simulink model "sst_llc_npc_inv"  (R2025b)
settings: Solver=ode23tb  StartTime=0.0  StopTime=simlength  FixedStep=tc  MaxStep=tc
values from neighbouring files (symbols this model uses):
  Adrso = eye(2) + Arso*ts_inv    [init_model.m]
  Aresd_max = eye(2) + Ares_max*ts_afe    [init_model.m]
  Aresd_min = eye(2) + Ares_min*ts_afe    [init_model.m]
  Aresd_nom = eye(2) + Ares_nom*ts_afe    [init_model.m]
  Bresd = Bres*ts_afe    [init_model.m]
  CFi_dc2 = 900e-6*4    (= 0.0036)    [init_model.m]
  Cresd = Cres    [init_model.m]
  Crso = [1 0]    [init_model.m]
  delta = 0.025    [init_model.m]
  fPWM_DAB = fPWM*4    (= 20000)    [init_model.m]
  freq = 50    [init_model.m]
  Iac_FS = I_phase_normalization_factor    [init_model.m]
  Idc_FS = max(Idab1_dc_nom,Idab2_dc_nom) * margin_factor    [init_model.m]
  iph_grid_pu_ref = 3.75    [init_model.m]
  ki_afe = 18    [init_model.m]
  ki_i_dab = 18    [init_model.m]
  ki_pll = 3140    [init_model.m]
  ki_rpi = 18    [init_model.m]
  kp_afe = 0.25    [init_model.m]
  kp_i_dab = 0.25    [init_model.m]
  kp_pll = 314    [init_model.m]
  kp_rpi = 0.25    [init_model.m]
  Ldrso = acker(Adrso',Crso',polesdrso)'    [init_model.m]
  LFu1_AFE = 0.33e-3    (= 0.00033)    [init_model.m]
  n_modules = 1    [init_model.m]
  RLFu1_AFE = 157*0.05*LFu1_AFE    (= 0.0025905)    [init_model.m]
  tc = ts_dab/1000*24    (= 1.2e-06)    [init_model.m]
  ts_afe = 1/fPWM_AFE    (= 0.0002)    [init_model.m]
  ts_dab = 1/fPWM_DAB    (= 5e-05)    [init_model.m]
  ts_inv = 1/fPWM_INV    (= 0.0002)    [init_model.m]
  Vac_FS = V_phase_normalization_factor    [init_model.m]
  Vdab2_dc_nom = 1500    [init_model.m]
  Vdc_FS = max(Vdab1_dc_nom,Vdab2_dc_nom) * margin_factor    [init_model.m]
undefined symbols (not defined in the file or in its folder): omega_grid_nom, V_phase_normalization_factor
libraries: fl_lib x68, nesl_utility x40, discrete_time_low_pass_filter x4, full_bridge_mosfet_based_with_thermal_model x2, single_phase_transformer x2, pi_ctrl x2, resonant_llc_modulator x2, full_bridge_ideal_switch x2, dclink_for_three_levels x2, full_bridge_three_level_npc_ideal_switch_based_model x2, single_phase_three_levels_PWM_modulator x2, dq_vector_pi x2
(part 2 of 4)

== system sst_llc_npc_inv/global timing/time_afe1 ==
  correction_time : Inport
  Constant : Constant
  Gain : Gain  Gain=k
  Product : Product
  Sum : Sum  Inputs=|++
  time_1 : Clock
  Out1 : Outport
  wires:
  time_1/1 -> Gain/1
  Gain/1 -> Product/1
  Product/1 -> Out1/1
  correction_time/1 -> Sum/1
  Sum/1 -> Product/2
  Constant/1 -> Sum/2

== system sst_llc_npc_inv/global timing/time_afe2 ==
  correction_time : Inport
  Constant : Constant
  Gain : Gain  Gain=k
  Product : Product
  Sum : Sum  Inputs=|++
  time_1 : Clock
  Out1 : Outport
  wires:
  time_1/1 -> Gain/1
  Gain/1 -> Product/1
  Product/1 -> Out1/1
  correction_time/1 -> Sum/1
  Constant/1 -> Sum/2
  Sum/1 -> Product/2

== system sst_llc_npc_inv/global timing/time_afe3 ==
  Gain : Gain  Gain=k
  time_1 : Clock
  Out1 : Outport
  wires:
  Gain/1 -> Out1/1
  time_1/1 -> Gain/1

== system sst_llc_npc_inv/global timing/time_inv1 ==
  correction_time : Inport
  Constant : Constant
  Gain : Gain  Gain=k
  Product : Product
  Sum : Sum  Inputs=|++
  time_1 : Clock
  Out1 : Outport
  wires:
  time_1/1 -> Gain/1
  Gain/1 -> Product/1
  Product/1 -> Out1/1
  correction_time/1 -> Sum/1
  Constant/1 -> Sum/2
  Sum/1 -> Product/2

== system sst_llc_npc_inv/global timing/time_inv2 ==
  correction_time : Inport
  Constant : Constant
  Gain : Gain  Gain=k
  Product : Product
  Sum : Sum  Inputs=|++
  time_1 : Clock
  Out1 : Outport
  wires:
  time_1/1 -> Gain/1
  Gain/1 -> Product/1
  Product/1 -> Out1/1
  correction_time/1 -> Sum/1
  Constant/1 -> Sum/2
  Sum/1 -> Product/2

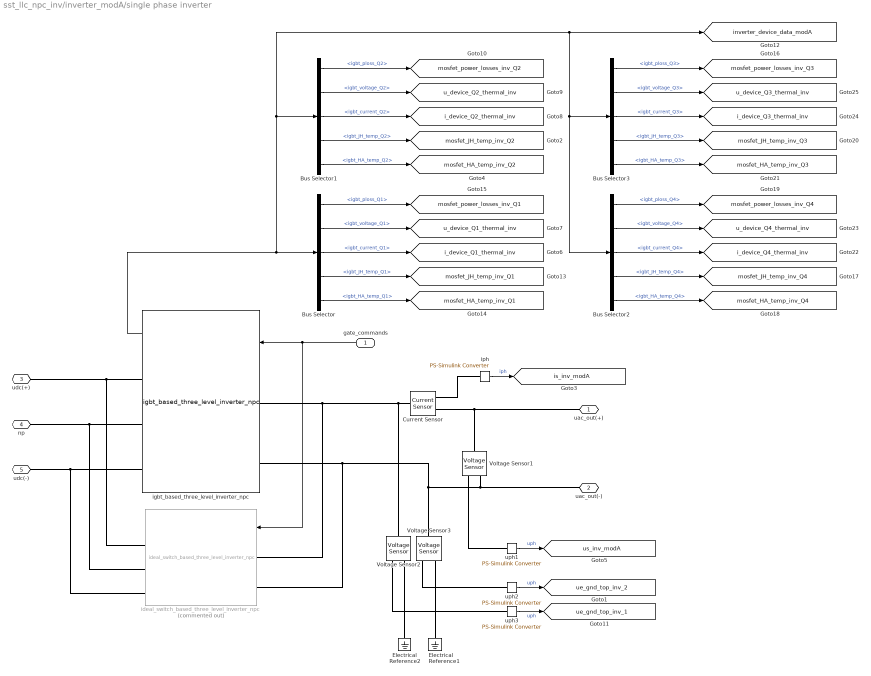
== system sst_llc_npc_inv/inverter_modA/single phase inverter ==
  gate_commands : Inport
  Bus Selector : BusSelector  OutputSignals=igbt_ploss_Q1,igbt_voltage_Q1,igbt_current_Q1,igbt_JH_temp_Q1,igbt_HA_temp_Q1
  Bus Selector1 : BusSelector  OutputSignals=igbt_ploss_Q2,igbt_voltage_Q2,igbt_current_Q2,igbt_JH_temp_Q2,igbt_HA_temp_Q2
  Bus Selector2 : BusSelector  OutputSignals=igbt_ploss_Q4,igbt_voltage_Q4,igbt_current_Q4,igbt_JH_temp_Q4,igbt_HA_temp_Q4
  Bus Selector3 : BusSelector  OutputSignals=igbt_ploss_Q3,igbt_voltage_Q3,igbt_current_Q3,igbt_JH_temp_Q3,igbt_HA_temp_Q3
  Current Sensor : fl_lib/Electrical/Electrical Sensors/Current Sensor
  Electrical Reference1 : fl_lib/Electrical/Electrical Elements/Electrical Reference
  Electrical Reference2 : fl_lib/Electrical/Electrical Elements/Electrical Reference
  Voltage Sensor1 : fl_lib/Electrical/Electrical Sensors/Voltage Sensor
  Voltage Sensor2 : fl_lib/Electrical/Electrical Sensors/Voltage Sensor
  Voltage Sensor3 : fl_lib/Electrical/Electrical Sensors/Voltage Sensor
  ideal_switch_based_three_level_inverter_npc : full_bridge_three_level_npc_ideal_switch_based_model/ideal_switch_based_three_level_inverter_npc  Commented=on  Vth=5.5  Ron=1.5e-3  Vdon_diode=1.65  Rdon_diode=0.15e-3  Csnubber=1e-10  Rsnubber=2200
  igbt_based_three_level_inverter_npc : full_bridge_three_level_npc_igbt_based_model/igbt_based_three_level_inverter_npc  Vth=inv.Vth  Vce_sat=inv.Vce_sat  Rce_on=inv.Rce_on  Eon=inv.Eon  Eoff=inv.Eoff  Erec=inv.Erec  Ion_sw_loss=inv.Ion_sw_losses  Voff_sw_loss=inv.Voff_sw_losses  Vdon_diode=inv.Vdon_diode  Rdon_diode=inv.Rdon_diode  rth_mosfet_JH=inv.Rth_switch_JH  rth_mosfet_HA=Rth_switch_HA  Csnubber=inv.Csnubber  Rsnubber=inv.Rsnubber  JunctionTermalMass=JunctionTermalMass  mass_heatsink=weigth  specific_heat=cp_al  Tambient=Tambient  DThs_init=DThs_init  tc=tc
  iph : nesl_utility/PS-Simulink Converter  PhysicalDomain=network_engine_domain  SubClassName=ps_output  LeftPortType=input  RightPortType=output  PseudoPeriodic=off  Frequencies=[]  VectorFormat=1-D array  Unit=A  AffineConversion=off
  uph1 : nesl_utility/PS-Simulink Converter  PhysicalDomain=network_engine_domain  SubClassName=ps_output  LeftPortType=input  RightPortType=output  PseudoPeriodic=off  Frequencies=[]  VectorFormat=1-D array  Unit=V  AffineConversion=off
  uph2 : nesl_utility/PS-Simulink Converter  PhysicalDomain=network_engine_domain  SubClassName=ps_output  LeftPortType=input  RightPortType=output  PseudoPeriodic=off  Frequencies=[]  VectorFormat=1-D array  Unit=V  AffineConversion=off
  uph3 : nesl_utility/PS-Simulink Converter  PhysicalDomain=network_engine_domain  SubClassName=ps_output  LeftPortType=input  RightPortType=output  PseudoPeriodic=off  Frequencies=[]  VectorFormat=1-D array  Unit=V  AffineConversion=off
  uac_out(+) : PMIOPort  Side=Left
  uac_out(-) : PMIOPort  Port=2  Side=Left
  udc(+) : PMIOPort  Port=3  Side=Right
  np : PMIOPort  Port=4  Side=Right
  udc(-) : PMIOPort  Port=5  Side=Right
  tag scope: i_device_Q1_thermal_inv=global, i_device_Q2_thermal_inv=global, i_device_Q3_thermal_inv=global, i_device_Q4_thermal_inv=global, inverter_device_data_modA=global, is_inv_modA=global, mosfet_HA_temp_inv_Q1=global, mosfet_HA_temp_inv_Q2=global, mosfet_HA_temp_inv_Q3=global, mosfet_HA_temp_inv_Q4=global, mosfet_JH_temp_inv_Q1=global, mosfet_JH_temp_inv_Q2=global, mosfet_JH_temp_inv_Q3=global, mosfet_JH_temp_inv_Q4=global, mosfet_power_losses_inv_Q1=global, mosfet_power_losses_inv_Q2=global, mosfet_power_losses_inv_Q3=global, mosfet_power_losses_inv_Q4=global, u_device_Q1_thermal_inv=global, u_device_Q2_thermal_inv=global, u_device_Q3_thermal_inv=global, u_device_Q4_thermal_inv=global, ue_gnd_top_inv_1=global, ue_gnd_top_inv_2=global, us_inv_modA=global
  wires:
  iph/1 -> [is_inv_modA]  "iph"
  uph1/1 -> [us_inv_modA]  "uph"
  gate_commands/1 -> ideal_switch_based_three_level_inverter_npc/1, igbt_based_three_level_inverter_npc/1
  Bus Selector/1 -> [mosfet_power_losses_inv_Q1]  "<igbt_ploss_Q1>"
  Bus Selector/2 -> [u_device_Q1_thermal_inv]  "<igbt_voltage_Q1>"
  Bus Selector/3 -> [i_device_Q1_thermal_inv]  "<igbt_current_Q1>"
  Bus Selector/4 -> [mosfet_JH_temp_inv_Q1]  "<igbt_JH_temp_Q1>"
  Bus Selector/5 -> [mosfet_HA_temp_inv_Q1]  "<igbt_HA_temp_Q1>"
  Bus Selector1/4 -> [mosfet_JH_temp_inv_Q2]  "<igbt_JH_temp_Q2>"
  Bus Selector1/5 -> [mosfet_HA_temp_inv_Q2]  "<igbt_HA_temp_Q2>"
  Bus Selector1/3 -> [i_device_Q2_thermal_inv]  "<igbt_current_Q2>"
  Bus Selector1/2 -> [u_device_Q2_thermal_inv]  "<igbt_voltage_Q2>"
  Bus Selector1/1 -> [mosfet_power_losses_inv_Q2]  "<igbt_ploss_Q2>"
  uph2/1 -> [ue_gnd_top_inv_2]  "uph"
  uph3/1 -> [ue_gnd_top_inv_1]  "uph"
  igbt_based_three_level_inverter_npc/1 -> Bus Selector2/1, Bus Selector3/1, [inverter_device_data_modA], Bus Selector1/1, Bus Selector/1
  Bus Selector3/1 -> [mosfet_power_losses_inv_Q3]  "<igbt_ploss_Q3>"
  Bus Selector3/2 -> [u_device_Q3_thermal_inv]  "<igbt_voltage_Q3>"
  Bus Selector3/3 -> [i_device_Q3_thermal_inv]  "<igbt_current_Q3>"
  Bus Selector3/5 -> [mosfet_HA_temp_inv_Q3]  "<igbt_HA_temp_Q3>"
  Bus Selector3/4 -> [mosfet_JH_temp_inv_Q3]  "<igbt_JH_temp_Q3>"
  Bus Selector2/5 -> [mosfet_HA_temp_inv_Q4]  "<igbt_HA_temp_Q4>"
  Bus Selector2/4 -> [mosfet_JH_temp_inv_Q4]  "<igbt_JH_temp_Q4>"
  Bus Selector2/3 -> [i_device_Q4_thermal_inv]  "<igbt_current_Q4>"
  Bus Selector2/2 -> [u_device_Q4_thermal_inv]  "<igbt_voltage_Q4>"
  Bus Selector2/1 -> [mosfet_power_losses_inv_Q4]  "<igbt_ploss_Q4>"
  connections:
  Current Sensor/RConn1 -- iph/LConn1
  Current Sensor/RConn2 -- Voltage Sensor1/LConn1 -- uac_out(+)/RConn1
  Voltage Sensor1/RConn1 -- uph1/LConn1
  Voltage Sensor1/RConn2 -- ideal_switch_based_three_level_inverter_npc/LConn2 -- igbt_based_three_level_inverter_npc/LConn2 -- Voltage Sensor3/LConn1 -- uac_out(-)/RConn1
  igbt_based_three_level_inverter_npc/RConn1 -- ideal_switch_based_three_level_inverter_npc/RConn1 -- udc(+)/RConn1
  Current Sensor/LConn1 -- ideal_switch_based_three_level_inverter_npc/LConn1 -- igbt_based_three_level_inverter_npc/LConn1 -- Voltage Sensor2/LConn1
  igbt_based_three_level_inverter_npc/RConn3 -- ideal_switch_based_three_level_inverter_npc/RConn3 -- udc(-)/RConn1
  Electrical Reference2/LConn1 -- Voltage Sensor2/RConn2
  Electrical Reference1/LConn1 -- Voltage Sensor3/RConn2
  uph2/LConn1 -- Voltage Sensor3/RConn1
  uph3/LConn1 -- Voltage Sensor2/RConn1
  igbt_based_three_level_inverter_npc/RConn2 -- ideal_switch_based_three_level_inverter_npc/RConn2 -- np/RConn1

== system sst_llc_npc_inv/inverter_modA/single phase inverter control1 ==
  Constant : Constant
  acquisition_and_scaling_current : Subsystem
  acquisition_and_scaling_dc_voltage : Subsystem
  acquisition_and_scaling_voltage : Subsystem
  acquisition_and_scaling_voltage1 : Subsystem
  inverter_current_output_pu_reference : Subsystem
  pwm modulator : Subsystem
  rpi_based_single_phase_inverter_ctrl : Subsystem
  gate_cmds : Outport
  u_ctrl_out : Outport  Port=2
  tag scope: phase_synch_modA=global
  wires:
  [is_inv_modA] -> acquisition_and_scaling_current/1(in)
  pwm modulator/1(gate_cmds) -> gate_cmds/1
  [TRGO_INV_1] -> rpi_based_single_phase_inverter_ctrl/Trigger
  [inverter_voltage_output_modA] -> acquisition_and_scaling_voltage/1(in)
  acquisition_and_scaling_current/1(out) -> rpi_based_single_phase_inverter_ctrl/2(is_inv_pu)  "is_inv_pu"
  acquisition_and_scaling_voltage/1(out) -> rpi_based_single_phase_inverter_ctrl/1(inverter_voltage_output_pu)  "inverter_voltage_output_pu"
  inverter_current_output_pu_reference/1(inverter_current_output_pu_reference) -> rpi_based_single_phase_inverter_ctrl/3(is_inv_pu_reference)  "inverter_current_output_pu_reference"
  [dclink_voltage_inverter_modA] -> acquisition_and_scaling_dc_voltage/1(in)
  rpi_based_single_phase_inverter_ctrl/1(u_ctrl_out) -> u_ctrl_out/1, pwm modulator/1(vout)
  acquisition_and_scaling_voltage1/1(out) -> rpi_based_single_phase_inverter_ctrl/5(u_line_pu)  "ac_grid_voltage_pu"
  [ac_grid_voltage] -> acquisition_and_scaling_voltage1/1(in)
  rpi_based_single_phase_inverter_ctrl/2(phase_grid_modA) -> [phase_synch_modA]
  [time_afe_module_1] -> rpi_based_single_phase_inverter_ctrl/6(time_afe_module_1)  "time_afe_module_1"
  Constant/1 -> rpi_based_single_phase_inverter_ctrl/4(dclink_voltage_pu)

== system sst_llc_npc_inv/inverter_modB/single phase inverter ==
  gate_commands : Inport
  Bus Selector : BusSelector  OutputSignals=switch_voltage_Q1,switch_current_Q1
  Current Sensor : fl_lib/Electrical/Electrical Sensors/Current Sensor
  Electrical Reference1 : fl_lib/Electrical/Electrical Elements/Electrical Reference
  Electrical Reference2 : fl_lib/Electrical/Electrical Elements/Electrical Reference
  Voltage Sensor1 : fl_lib/Electrical/Electrical Sensors/Voltage Sensor
  Voltage Sensor2 : fl_lib/Electrical/Electrical Sensors/Voltage Sensor
  Voltage Sensor3 : fl_lib/Electrical/Electrical Sensors/Voltage Sensor
  ideal_switch_based_three_level_inverter_npc : full_bridge_three_level_npc_ideal_switch_based_model/ideal_switch_based_three_level_inverter_npc  Vth=5.5  Ron=1.5e-3  Vdon_diode=1.65  Rdon_diode=0.15e-3  Csnubber=1e-10  Rsnubber=2200
  iph : nesl_utility/PS-Simulink Converter  PhysicalDomain=network_engine_domain  SubClassName=ps_output  LeftPortType=input  RightPortType=output  PseudoPeriodic=off  Frequencies=[]  VectorFormat=1-D array  Unit=A  AffineConversion=off
  uph1 : nesl_utility/PS-Simulink Converter  PhysicalDomain=network_engine_domain  SubClassName=ps_output  LeftPortType=input  RightPortType=output  PseudoPeriodic=off  Frequencies=[]  VectorFormat=1-D array  Unit=V  AffineConversion=off
  uph2 : nesl_utility/PS-Simulink Converter  PhysicalDomain=network_engine_domain  SubClassName=ps_output  LeftPortType=input  RightPortType=output  PseudoPeriodic=off  Frequencies=[]  VectorFormat=1-D array  Unit=V  AffineConversion=off
  uph3 : nesl_utility/PS-Simulink Converter  PhysicalDomain=network_engine_domain  SubClassName=ps_output  LeftPortType=input  RightPortType=output  PseudoPeriodic=off  Frequencies=[]  VectorFormat=1-D array  Unit=V  AffineConversion=off
  uac_out(+) : PMIOPort  Side=Left
  uac_out(-) : PMIOPort  Port=2  Side=Left
  udc(+) : PMIOPort  Port=3  Side=Right
  np : PMIOPort  Port=4  Side=Right
  udc(-) : PMIOPort  Port=5  Side=Right
  tag scope: i_device_Q1_ideal_inv_modB=global, inverter_device_data_modB=global, is_inv_modB=global, u_device_Q1_ideal_inv_modB=global, ue_gnd_bottom_inv_1=global, ue_gnd_bottom_inv_2=global, us_inv_modB=global
  wires:
  gate_commands/1 -> ideal_switch_based_three_level_inverter_npc/1
  uph1/1 -> [us_inv_modB]  "uph"
  iph/1 -> [is_inv_modB]  "iph"
  uph3/1 -> [ue_gnd_bottom_inv_1]  "uph"
  uph2/1 -> [ue_gnd_bottom_inv_2]  "uph"
  ideal_switch_based_three_level_inverter_npc/1 -> Bus Selector/1, [inverter_device_data_modB]
  Bus Selector/2 -> [i_device_Q1_ideal_inv_modB]  "<switch_current_Q1>"
  Bus Selector/1 -> [u_device_Q1_ideal_inv_modB]  "<switch_voltage_Q1>"
  connections:
  ideal_switch_based_three_level_inverter_npc/RConn3 -- udc(-)/RConn1
  Voltage Sensor2/LConn1 -- ideal_switch_based_three_level_inverter_npc/LConn1 -- Current Sensor/LConn1
  ideal_switch_based_three_level_inverter_npc/RConn1 -- udc(+)/RConn1
  uac_out(-)/RConn1 -- ideal_switch_based_three_level_inverter_npc/LConn2 -- Voltage Sensor3/LConn1 -- Voltage Sensor1/RConn2
  Voltage Sensor1/RConn1 -- uph1/LConn1
  uac_out(+)/RConn1 -- Voltage Sensor1/LConn1 -- Current Sensor/RConn2
  Current Sensor/RConn1 -- iph/LConn1
  Electrical Reference2/LConn1 -- Voltage Sensor2/RConn2
  uph2/LConn1 -- Voltage Sensor3/RConn1
  uph3/LConn1 -- Voltage Sensor2/RConn1
  Electrical Reference1/LConn1 -- Voltage Sensor3/RConn2
  ideal_switch_based_three_level_inverter_npc/RConn2 -- np/RConn1

== system sst_llc_npc_inv/inverter_modB/single phase inverter control1 ==
  acquisition_and_scaling_current : Subsystem
  acquisition_and_scaling_dc_voltage : Subsystem
  acquisition_and_scaling_voltage : Subsystem
  acquisition_and_scaling_voltage1 : Subsystem
  inverter_current_output_pu_reference : Subsystem
  pwm modulator : Subsystem
  rpi_based_single_phase_inverter_ctrl : Subsystem
  gate_cmds : Outport
  tag scope: phase_synch_modB=global
  wires:
  pwm modulator/1(gate_cmds) -> gate_cmds/1
  rpi_based_single_phase_inverter_ctrl/2(phase_grid_modA) -> [phase_synch_modB]
  rpi_based_single_phase_inverter_ctrl/1(u_ctrl_out) -> pwm modulator/1(vout)
  [u_ctrl_out_master] -> rpi_based_single_phase_inverter_ctrl/6(u_ctrl_out_master)  "u_ctrl_out_master"
  acquisition_and_scaling_dc_voltage/1(out) -> rpi_based_single_phase_inverter_ctrl/4(dclink_voltage_pu)
  acquisition_and_scaling_voltage1/1(out) -> rpi_based_single_phase_inverter_ctrl/5(u_line_pu)  "u_line_pu"
  acquisition_and_scaling_current/1(out) -> rpi_based_single_phase_inverter_ctrl/2(is_inv_pu)  "is_inv_pu"
  [inverter_voltage_output_modB] -> acquisition_and_scaling_voltage/1(in)
  [ac_grid_voltage] -> acquisition_and_scaling_voltage1/1(in)
  acquisition_and_scaling_voltage/1(out) -> rpi_based_single_phase_inverter_ctrl/1(inverter_voltage_output_pu)  "inverter_voltage_output_pu"
  [dclink_voltage_inverter_modB] -> acquisition_and_scaling_dc_voltage/1(in)
  [is_inv_modB] -> acquisition_and_scaling_current/1(in)
  inverter_current_output_pu_reference/1(inverter_current_output_pu_reference) -> rpi_based_single_phase_inverter_ctrl/3(is_inv_pu_reference)  "inverter_current_output_pu_reference"
  [TRGO_INV_2] -> rpi_based_single_phase_inverter_ctrl/Trigger

== system sst_llc_npc_inv/line_source/phase_gen ==
  Constant4 : Constant  Value=50*2*pi
  Integrator : Integrator
  bounder1 : MATLAB Function  TreatAsAtomicUnit=on
  phase_gen : Outport  VectorParamsAs1DForOutWhenUnconnected=off
  wires:
  Constant4/1 -> Integrator/1
  Integrator/1 -> bounder1/1(u)
  bounder1/1(y) -> phase_gen/1  "grid_emu_phase"

== system sst_llc_npc_inv/scopes/scopes_dab_modA ==
  Bus Selector : BusSelector  OutputSignals=mosfet_ploss_Q1,mosfet_ploss_Q2
  Bus Selector1 : BusSelector  OutputSignals=mosfet_ploss_Q1,mosfet_ploss_Q2
  dab TR i2/i1 modA : Scope  NumInputPorts=2
      settings: SampleTime=tc  ActiveDisplayYMinimum=-1515.8601129634949  ActiveDisplayYMaximum=1519.4045908602914  DataLoggingVariableName=ScopeData13
  dab TR u2/u1 modA : Scope  NumInputPorts=2
      settings: SampleTime=tc  ActiveDisplayYMinimum=-893.62031856834165  ActiveDisplayYMaximum=653.92363611228757  DataLoggingVariableName=ScopeData4
  dab current output/input modA : Scope  NumInputPorts=2
      settings: SampleTime=tc  ActiveDisplayYMinimum=-34.407086049322743  ActiveDisplayYMaximum=284.20809963586862  DataLoggingVariableName=ScopeData8
  dab outputs modA : Scope  NumInputPorts=2
      settings: SampleTime=tc  ActiveDisplayYMinimum=-1504.2584903012705  ActiveDisplayYMaximum=905.23681286440785  DataLoggingVariableName=ScopeData6
  dab voltage input/output modA : Scope  NumInputPorts=2
      settings: SampleTime=tc  ActiveDisplayYMinimum=-224.45374462345234  ActiveDisplayYMaximum=1977.0471198962268  DataLoggingVariableName=ScopeData10
  dab_analysis_modA : Scope  NumInputPorts=4
      settings: SampleTime=tc  ActiveDisplayYMinimum=-1467.7661945335567  ActiveDisplayYMaximum=1564.8120287034021  DataLoggingVariableName=ScopeData15
  dab_analysis_power loss : Scope  NumInputPorts=4
      settings: SampleTime=tc  ActiveDisplayYMinimum=-26.281609666205206  ActiveDisplayYMaximum=283.03149514655593  DataLoggingVariableName=ScopeData17
  wires:
  [dab_voltage_input_modA] -> dab voltage input/output modA/1  "dab_voltage_input_modA"
  [dab_current_output_modA] -> dab current output/input modA/1  "dab_current_output_modA"
  [dab_voltage_output_modA] -> dab voltage input/output modA/2  "dab_voltage_output_modA"
  [dab_current_input_modA] -> dab current output/input modA/2  "dab_current_input_modA"
  [i2_dab_transformer_modA] -> dab TR i2/i1 modA/1  "i2_dab_transformer_modA"
  [i1_dab_transformer_modA] -> dab TR i2/i1 modA/2  "i1_dab_transformer_modA"
  [u2_dab_transformer_modA] -> dab TR u2/u1 modA/1  "u2_dab_transformer_modA"
  [u1_dab_transformer_modA] -> dab TR u2/u1 modA/2  "u1_dab_transformer_modA"
  [dab_voltage_output_modA] -> dab outputs modA/2  "dab_voltage_output_modA"
  [dab_current_output_modA] -> dab outputs modA/1  "dab_current_output_modA"
  [i2_dab_transformer_modA] -> dab_analysis_modA/1  "i2_dab_transformer_modA"
  [i1_dab_transformer_modA] -> dab_analysis_modA/2  "i1_dab_transformer_modA"
  [u1_dab_transformer_modA] -> dab_analysis_modA/3  "u1_dab_transformer_modA"
  [u2_dab_transformer_modA] -> dab_analysis_modA/4  "u2_dab_transformer_modA"
  [inverter_1_dab_devices_modA] -> Bus Selector/1
  [inverter_2_dab_devices_modA] -> Bus Selector1/1
  Bus Selector/1 -> dab_analysis_power loss/1  "<mosfet_ploss_Q1>"
  Bus Selector/2 -> dab_analysis_power loss/2  "<mosfet_ploss_Q2>"
  Bus Selector1/1 -> dab_analysis_power loss/3  "<mosfet_ploss_Q1>"
  Bus Selector1/2 -> dab_analysis_power loss/4  "<mosfet_ploss_Q2>"

== system sst_llc_npc_inv/scopes/scopes_dab_modB ==
  dab TR i2/i1 modB : Scope  NumInputPorts=2
      settings: SampleTime=tc  ActiveDisplayYMinimum=-700.08630880673149  ActiveDisplayYMaximum=469.74027472719069  DataLoggingVariableName=ScopeData13
  dab TR u2/u1 modB : Scope  NumInputPorts=2
      settings: SampleTime=tc  ActiveDisplayYMinimum=-893.62031856834165  ActiveDisplayYMaximum=653.92363611228757  DataLoggingVariableName=ScopeData4
  dab current output/input modB : Scope  NumInputPorts=2
      settings: SampleTime=tc  ActiveDisplayYMinimum=-7335.7913745283768  ActiveDisplayYMaximum=23819.434208451414  DataLoggingVariableName=ScopeData8
  dab outputs modB : Scope  NumInputPorts=2
      settings: SampleTime=tc  ActiveDisplayYMinimum=-1276.7812228163118  ActiveDisplayYMaximum=1202.3221787513703  DataLoggingVariableName=ScopeData6
  dab voltage input/output modB : Scope  NumInputPorts=2
      settings: SampleTime=tc  ActiveDisplayYMinimum=-237.60937353263552  ActiveDisplayYMaximum=2138.4843617937204  DataLoggingVariableName=ScopeData10
  dab_analysis_modB : Scope  NumInputPorts=4
      settings: SampleTime=tc  ActiveDisplayYMinimum=-1515.8601129634949  ActiveDisplayYMaximum=1519.4045908602914  DataLoggingVariableName=ScopeData15
  wires:
  [u2_dab_transformer_modB] -> dab_analysis_modB/4  "u2_dab_transformer_modB"
  [u1_dab_transformer_modB] -> dab_analysis_modB/3  "u1_dab_transformer_modB"
  [i1_dab_transformer_modB] -> dab_analysis_modB/2  "i1_dab_transformer_modB"
  [i2_dab_transformer_modB] -> dab_analysis_modB/1  "i2_dab_transformer_modB"
  [dab_current_output_modB] -> dab outputs modB/1  "dab_current_output_modB"
  [dab_voltage_output_modB] -> dab outputs modB/2  "dab_voltage_output_modB"
  [u1_dab_transformer_modB] -> dab TR u2/u1 modB/2  "u1_dab_transformer_modB"
  [u2_dab_transformer_modB] -> dab TR u2/u1 modB/1  "u2_dab_transformer_modB"
  [i1_dab_transformer_modB] -> dab TR i2/i1 modB/2  "i1_dab_transformer_modB"
  [i2_dab_transformer_modB] -> dab TR i2/i1 modB/1  "i2_dab_transformer_modB"
  [dab_current_input_modB] -> dab current output/input modB/2  "dab_current_input_modB"
  [dab_voltage_output_modB] -> dab voltage input/output modB/2  "dab_voltage_output_modB"
  [dab_current_output_modB] -> dab current output/input modB/1  "dab_current_output_modB"
  [dab_voltage_input_modB] -> dab voltage input/output modB/1  "dab_voltage_input_modB"

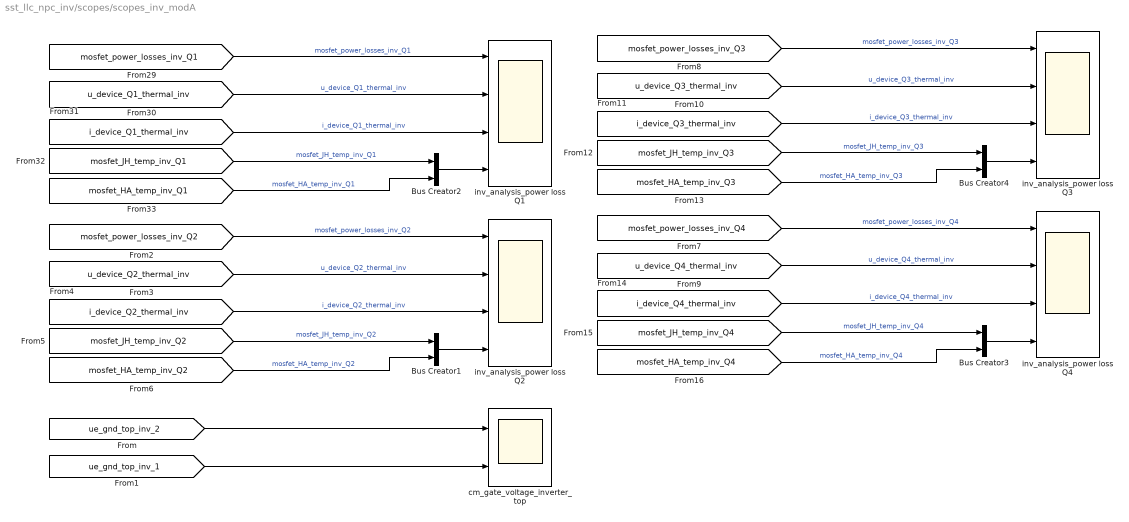
== system sst_llc_npc_inv/scopes/scopes_inv_modA ==
  Bus Creator{1..4} (4 alike) : BusCreator  Inputs=2
  cm_gate_voltage_inverter_top : Scope  NumInputPorts=2
      settings: SampleTime=tc  ActiveDisplayYMinimum=-1089.6954299405313  ActiveDisplayYMaximum=1165.8713445946826  DataLoggingVariableName=ScopeData22
  inv_analysis_power loss Q{1..4} (4 alike) : Scope  NumInputPorts=4
      inv_analysis_power loss Q1 settings: SampleTime=tc  ActiveDisplayYMinimum=252.03887543128099  ActiveDisplayYMaximum=654.5130246681365  DataLoggingVariableName=ScopeData18
      inv_analysis_power loss Q2 settings: SampleTime=tc  ActiveDisplayYMinimum=1215.5585157804567  ActiveDisplayYMaximum=1882.3509853926439  DataLoggingVariableName=ScopeData5
      inv_analysis_power loss Q3 settings: SampleTime=tc  ActiveDisplayYMinimum=1399.7218598743666  ActiveDisplayYMaximum=1614.3940109339064  DataLoggingVariableName=ScopeData16
      inv_analysis_power loss Q4 settings: SampleTime=tc  ActiveDisplayYMinimum=401.80036733196005  ActiveDisplayYMaximum=489.90080295034829  DataLoggingVariableName=ScopeData19
  wires:
  [mosfet_JH_temp_inv_Q1] -> Bus Creator2/1  "mosfet_JH_temp_inv_Q1"
  [u_device_Q1_thermal_inv] -> inv_analysis_power loss Q1/2  "u_device_Q1_thermal_inv"
  [i_device_Q1_thermal_inv] -> inv_analysis_power loss Q1/3  "i_device_Q1_thermal_inv"
  [mosfet_HA_temp_inv_Q1] -> Bus Creator2/2  "mosfet_HA_temp_inv_Q1"
  Bus Creator2/1 -> inv_analysis_power loss Q1/4
  [mosfet_power_losses_inv_Q1] -> inv_analysis_power loss Q1/1  "mosfet_power_losses_inv_Q1"
  [ue_gnd_top_inv_2] -> cm_gate_voltage_inverter_top/1
  [ue_gnd_top_inv_1] -> cm_gate_voltage_inverter_top/2
  [mosfet_power_losses_inv_Q2] -> inv_analysis_power loss Q2/1  "mosfet_power_losses_inv_Q2"
  Bus Creator1/1 -> inv_analysis_power loss Q2/4
  [mosfet_HA_temp_inv_Q2] -> Bus Creator1/2  "mosfet_HA_temp_inv_Q2"
  [i_device_Q2_thermal_inv] -> inv_analysis_power loss Q2/3  "i_device_Q2_thermal_inv"
  [u_device_Q2_thermal_inv] -> inv_analysis_power loss Q2/2  "u_device_Q2_thermal_inv"
  [mosfet_JH_temp_inv_Q2] -> Bus Creator1/1  "mosfet_JH_temp_inv_Q2"
  [mosfet_JH_temp_inv_Q4] -> Bus Creator3/1  "mosfet_JH_temp_inv_Q4"
  [u_device_Q4_thermal_inv] -> inv_analysis_power loss Q4/2  "u_device_Q4_thermal_inv"
  [i_device_Q4_thermal_inv] -> inv_analysis_power loss Q4/3  "i_device_Q4_thermal_inv"
  [mosfet_HA_temp_inv_Q4] -> Bus Creator3/2  "mosfet_HA_temp_inv_Q4"
  Bus Creator3/1 -> inv_analysis_power loss Q4/4
  [mosfet_power_losses_inv_Q4] -> inv_analysis_power loss Q4/1  "mosfet_power_losses_inv_Q4"
  [mosfet_power_losses_inv_Q3] -> inv_analysis_power loss Q3/1  "mosfet_power_losses_inv_Q3"
  Bus Creator4/1 -> inv_analysis_power loss Q3/4
  [mosfet_HA_temp_inv_Q3] -> Bus Creator4/2  "mosfet_HA_temp_inv_Q3"
  [i_device_Q3_thermal_inv] -> inv_analysis_power loss Q3/3  "i_device_Q3_thermal_inv"
  [u_device_Q3_thermal_inv] -> inv_analysis_power loss Q3/2  "u_device_Q3_thermal_inv"
  [mosfet_JH_temp_inv_Q3] -> Bus Creator4/1  "mosfet_JH_temp_inv_Q3"

== system sst_llc_npc_inv/scopes/scopes_inv_modB ==
  cm_gate_voltage_inverter_bottom : Scope  NumInputPorts=2
      settings: SampleTime=tc  ActiveDisplayYMinimum=-1241.6958905586757  ActiveDisplayYMaximum=1224.9152234663466  DataLoggingVariableName=ScopeData22
  device_voltage_current_inv Q1 modB : Scope  NumInputPorts=3
      settings: SampleTime=tc  ActiveDisplayYMinimum=-119.06518095025848  ActiveDisplayYMaximum=1054.0032225267662  DataLoggingVariableName=ScopeData20
  wires:
  [ue_gnd_bottom_inv_1] -> cm_gate_voltage_inverter_bottom/2
  [ue_gnd_bottom_inv_2] -> cm_gate_voltage_inverter_bottom/1
  [i_device_Q1_ideal_inv_modB] -> device_voltage_current_inv Q1 modB/2  "iQ1"
  [u_device_Q1_ideal_inv_modB] -> device_voltage_current_inv Q1 modB/1  "uQ1"
  [udc12_inverter_modB] -> device_voltage_current_inv Q1 modB/3  "udcs"

== system sst_llc_npc_inv/dcdc_llc_modA/dc//dc with galvanic isolation/full-bridge 1 ==
  gate_commands : Inport
  Bus Selector : BusSelector  OutputSignals=mosfet_ploss_Q1,mosfet_voltage_Q1,mosfet_current_Q1,mosfet_JH_temp_Q1,mosfet_HA_temp_Q1
  Bus Selector1 : BusSelector  OutputSignals=mosfet_ploss_Q2,mosfet_voltage_Q2,mosfet_current_Q2,mosfet_JH_temp_Q2,mosfet_HA_temp_Q2
  full-bridge mosfet based with thermal model : full_bridge_mosfet_based_with_thermal_model/full-bridge mosfet based with thermal model  mass_heatsink=weigth  specific_heat=cp_al  rth_mosfet_HA=Rth_mosfet_HA  rth_mosfet_JH=dab.Rth_mosfet_JH  Rds_on=dab.Rds_on  Vth=dab.Vth  Eon=dab.Eon  Eoff=dab.Eoff  Voff_sw_loss=dab.Voff_sw_losses  Ion_sw_loss=dab.Ion_sw_losses  Vdon_diode=dab.Vdon_diode  Rdon_diode=0.00185  JunctionTermalMass=JunctionTermalMass  Tambient=Tambient  DThs_init=DThs_init
  uac_1(+) : PMIOPort  Side=Left
  uac_1(-) : PMIOPort  Port=2  Side=Left
  Udc(+) : PMIOPort  Port=3  Side=Right
  Udc(-) : PMIOPort  Port=4  Side=Right
  tag scope: i_device_Q1_thermal_dab=global, i_device_Q2_thermal_dab=global, inverter_1_dab_devices_modA=global, mosfet_HA_temp_dab_Q1=global, mosfet_HA_temp_dab_Q2=global, mosfet_JH_temp_dab_Q1=global, mosfet_JH_temp_dab_Q2=global, mosfet_power_losses_dab_Q1=global, mosfet_power_losses_dab_Q2=global, u_device_Q1_thermal_dab=global, u_device_Q2_thermal_dab=global
  wires:
  gate_commands/1 -> full-bridge mosfet based with thermal model/1
  Bus Selector/1 -> [mosfet_power_losses_dab_Q1]  "<mosfet_ploss_Q1>"
  Bus Selector/2 -> [u_device_Q1_thermal_dab]  "<mosfet_voltage_Q1>"
  Bus Selector/3 -> [i_device_Q1_thermal_dab]  "<mosfet_current_Q1>"
  Bus Selector/4 -> [mosfet_JH_temp_dab_Q1]  "<mosfet_JH_temp_Q1>"
  Bus Selector/5 -> [mosfet_HA_temp_dab_Q1]  "<mosfet_HA_temp_Q1>"
  Bus Selector1/5 -> [mosfet_HA_temp_dab_Q2]  "<mosfet_HA_temp_Q2>"
  Bus Selector1/4 -> [mosfet_JH_temp_dab_Q2]  "<mosfet_JH_temp_Q2>"
  Bus Selector1/3 -> [i_device_Q2_thermal_dab]  "<mosfet_current_Q2>"
  Bus Selector1/2 -> [u_device_Q2_thermal_dab]  "<mosfet_voltage_Q2>"
  Bus Selector1/1 -> [mosfet_power_losses_dab_Q2]  "<mosfet_ploss_Q2>"
  full-bridge mosfet based with thermal model/1 -> [inverter_1_dab_devices_modA], Bus Selector1/1, Bus Selector/1
  connections:
  full-bridge mosfet based with thermal model/RConn1 -- uac_1(+)/RConn1
  full-bridge mosfet based with thermal model/RConn2 -- uac_1(-)/RConn1
  Udc(-)/RConn1 -- full-bridge mosfet based with thermal model/LConn2
  full-bridge mosfet based with thermal model/LConn1 -- Udc(+)/RConn1

== system sst_llc_npc_inv/dcdc_llc_modA/dc//dc with galvanic isolation/full-bridge 2 ==
  gate_commands : Inport
  Bus Selector : BusSelector  OutputSignals=mosfet_ploss_Q1,mosfet_voltage_Q1,mosfet_current_Q1,mosfet_JH_temp_Q1,mosfet_HA_temp_Q1
  Bus Selector1 : BusSelector  OutputSignals=mosfet_ploss_Q2,mosfet_voltage_Q2,mosfet_current_Q2,mosfet_JH_temp_Q2,mosfet_HA_temp_Q2
  CFi_dc2 : fl_lib/Electrical/Electrical Elements/Capacitor  c=CFi_dc2 F  r=RCFi_dc2_internal Ohm  g=0 1/Ohm  i_specify=off  i_priority=None  i=0 A  i_nominal_specify=off  i_nominal_value=1  i_nominal_unit=A  v_specify=off  v_priority=None  v=0 V  v_nominal_specify=off  v_nominal_value=1  v_nominal_unit=V  vc_specify=off  vc_priority=High  vc=0 V  vc_nominal_specify=off  vc_nominal_value=1  vc_nominal_unit=V
  Current Sensor2 : fl_lib/Electrical/Electrical Sensors/Current Sensor
  PS-Simulink Converter6 : nesl_utility/PS-Simulink Converter  PhysicalDomain=network_engine_domain  SubClassName=ps_output  LeftPortType=input  RightPortType=output  PseudoPeriodic=off  Frequencies=[]  VectorFormat=1-D array  Unit=A  AffineConversion=on
  full-bridge mosfet based with thermal model : full_bridge_mosfet_based_with_thermal_model/full-bridge mosfet based with thermal model  mass_heatsink=weigth  specific_heat=cp_al  rth_mosfet_HA=Rth_mosfet_HA  rth_mosfet_JH=dab.Rth_mosfet_JH  Rds_on=dab.Rds_on  Vth=dab.Vth  Eon=dab.Eon  Eoff=dab.Eoff  Voff_sw_loss=dab.Voff_sw_losses  Ion_sw_loss=dab.Ion_sw_losses  Vdon_diode=dab.Vdon_diode  Rdon_diode=0.00185  JunctionTermalMass=JunctionTermalMass  Tambient=Tambient  DThs_init=DThs_init
  uac_2(+) : PMIOPort  Side=Left
  uac_2(-) : PMIOPort  Port=2  Side=Left
  udc(+) : PMIOPort  Port=3  Side=Right
  udc(-) : PMIOPort  Port=4  Side=Right
  tag scope: CFi_dc2_current_modA=global, i_device_Q5_thermal_dab=global, i_device_Q6_thermal_dab=global, inverter_2_dab_devices_modA=global, mosfet_HA_temp_dab_Q5=global, mosfet_HA_temp_dab_Q6=global, mosfet_JH_temp_dab_Q5=global, mosfet_JH_temp_dab_Q6=global, mosfet_power_losses_dab_Q5=global, mosfet_power_losses_dab_Q6=global, u_device_Q5_thermal_dab=global, u_device_Q6_thermal_dab=global
  wires:
  gate_commands/1 -> full-bridge mosfet based with thermal model/1
  PS-Simulink Converter6/1 -> [CFi_dc2_current_modA]  "CFi_dc2_current_modA"
  Bus Selector/4 -> [mosfet_JH_temp_dab_Q5]  "<mosfet_JH_temp_Q1>"
  Bus Selector/3 -> [i_device_Q5_thermal_dab]  "<mosfet_current_Q1>"
  Bus Selector/5 -> [mosfet_HA_temp_dab_Q5]  "<mosfet_HA_temp_Q1>"
  Bus Selector/1 -> [mosfet_power_losses_dab_Q5]  "<mosfet_ploss_Q1>"
  Bus Selector/2 -> [u_device_Q5_thermal_dab]  "<mosfet_voltage_Q1>"
  full-bridge mosfet based with thermal model/1 -> [inverter_2_dab_devices_modA], Bus Selector1/1, Bus Selector/1
  Bus Selector1/2 -> [u_device_Q6_thermal_dab]  "<mosfet_voltage_Q2>"
  Bus Selector1/1 -> [mosfet_power_losses_dab_Q6]  "<mosfet_ploss_Q2>"
  Bus Selector1/5 -> [mosfet_HA_temp_dab_Q6]  "<mosfet_HA_temp_Q2>"
  Bus Selector1/3 -> [i_device_Q6_thermal_dab]  "<mosfet_current_Q2>"
  Bus Selector1/4 -> [mosfet_JH_temp_dab_Q6]  "<mosfet_JH_temp_Q2>"
  connections:
  udc(+)/RConn1 -- full-bridge mosfet based with thermal model/LConn1 -- CFi_dc2/LConn1
  Current Sensor2/RConn2 -- full-bridge mosfet based with thermal model/LConn2 -- udc(-)/RConn1
  PS-Simulink Converter6/LConn1 -- Current Sensor2/RConn1
  CFi_dc2/RConn1 -- Current Sensor2/LConn1
  full-bridge mosfet based with thermal model/RConn1 -- uac_2(+)/RConn1
  full-bridge mosfet based with thermal model/RConn2 -- uac_2(-)/RConn1

== system sst_llc_npc_inv/dcdc_llc_modA/dc//dc with galvanic isolation/single_phase_dab_transformer ==
  Capacitor : fl_lib/Electrical/Electrical Elements/Capacitor  c=Cs1 F  r=1e-6 Ohm  g=0 1/Ohm  i_specify=off  i_priority=None  i=0 A  i_nominal_specify=off  i_nominal_value=1  i_nominal_unit=A  v_specify=off  v_priority=None  v=0 V  v_nominal_specify=off  v_nominal_value=1  v_nominal_unit=V  vc_specify=off  vc_priority=High  vc=0 V  vc_nominal_specify=off  vc_nominal_value=1  vc_nominal_unit=V
  Capacitor1 : fl_lib/Electrical/Electrical Elements/Capacitor  c=Cs2 F  r=1e-6 Ohm  g=0 1/Ohm  i_specify=off  i_priority=None  i=0 A  i_nominal_specify=off  i_nominal_value=1  i_nominal_unit=A  v_specify=off  v_priority=None  v=0 V  v_nominal_specify=off  v_nominal_value=1  v_nominal_unit=V  vc_specify=off  vc_priority=High  vc=0 V  vc_nominal_specify=off  vc_nominal_value=1  vc_nominal_unit=V
  Current Sensor : fl_lib/Electrical/Electrical Sensors/Current Sensor
  Current Sensor1 : fl_lib/Electrical/Electrical Sensors/Current Sensor
  Voltage Sensor1 : fl_lib/Electrical/Electrical Sensors/Voltage Sensor
  Voltage Sensor3 : fl_lib/Electrical/Electrical Sensors/Voltage Sensor
  i1_dab_transformer : nesl_utility/PS-Simulink Converter  PhysicalDomain=network_engine_domain  SubClassName=ps_output  LeftPortType=input  RightPortType=output  PseudoPeriodic=off  Frequencies=[]  VectorFormat=1-D array  Unit=A  AffineConversion=off
  i2_dab_transformer : nesl_utility/PS-Simulink Converter  PhysicalDomain=network_engine_domain  SubClassName=ps_output  LeftPortType=input  RightPortType=output  PseudoPeriodic=off  Frequencies=[]  VectorFormat=1-D array  Unit=A  AffineConversion=off
  single_phase_transformer : single_phase_transformer/single_phase_transformer  lm_trafo=lm_trafo  m1=m1  m2=m2  rd1_trafo=rd1_trafo  rd2_trafo=rd2_trafo  ld1_trafo=ld1_trafo  ld2_trafo=ld2_trafo  rfe_trafo=rfe_trafo  length_core=0.5  mu0=1.256637e-6  mur=70
  single_phase_transformer - scope : Scope
      settings: ActiveDisplayYMinimum=-1507.7800736606021  ActiveDisplayYMaximum=1558.2525629015804  DataLoggingVariableName=ScopeData21
  u1_dab_transformer : nesl_utility/PS-Simulink Converter  PhysicalDomain=network_engine_domain  SubClassName=ps_output  LeftPortType=input  RightPortType=output  PseudoPeriodic=off  Frequencies=[]  VectorFormat=1-D array  Unit=V  AffineConversion=on
  u2_dab_transformer : nesl_utility/PS-Simulink Converter  PhysicalDomain=network_engine_domain  SubClassName=ps_output  LeftPortType=input  RightPortType=output  PseudoPeriodic=off  Frequencies=[]  VectorFormat=1-D array  Unit=V  AffineConversion=on
  u1(+) : PMIOPort  Side=Left
  u2(+) : PMIOPort  Port=2  Side=Right
  u1(-) : PMIOPort  Port=3  Side=Left
  u2(-) : PMIOPort  Port=4  Side=Right
  tag scope: i1_dab_transformer_modA=global, i2_dab_transformer_modA=global, u1_dab_transformer_modA=global, u2_dab_transformer_modA=global
  wires:
  i2_dab_transformer/1 -> [i2_dab_transformer_modA]
  u2_dab_transformer/1 -> [u2_dab_transformer_modA]
  u1_dab_transformer/1 -> [u1_dab_transformer_modA]
  i1_dab_transformer/1 -> [i1_dab_transformer_modA]
  single_phase_transformer/1 -> single_phase_transformer - scope/1
  connections:
  Current Sensor/RConn2 -- u2(+)/RConn1
  Voltage Sensor3/RConn2 -- single_phase_transformer/RConn2 -- u2(-)/RConn1
  Current Sensor/RConn1 -- i2_dab_transformer/LConn1
  Voltage Sensor3/RConn1 -- u2_dab_transformer/LConn1
  u1(-)/RConn1 -- single_phase_transformer/LConn2 -- Voltage Sensor1/RConn2
  Current Sensor1/LConn1 -- Voltage Sensor1/LConn1 -- u1(+)/RConn1
  Voltage Sensor1/RConn1 -- u1_dab_transformer/LConn1
  Current Sensor1/RConn1 -- i1_dab_transformer/LConn1
  Voltage Sensor3/LConn1 -- Capacitor1/RConn1 -- Current Sensor/LConn1
  single_phase_transformer/LConn1 -- Capacitor/RConn1
  Capacitor/LConn1 -- Current Sensor1/RConn2
  single_phase_transformer/RConn1 -- Capacitor1/LConn1

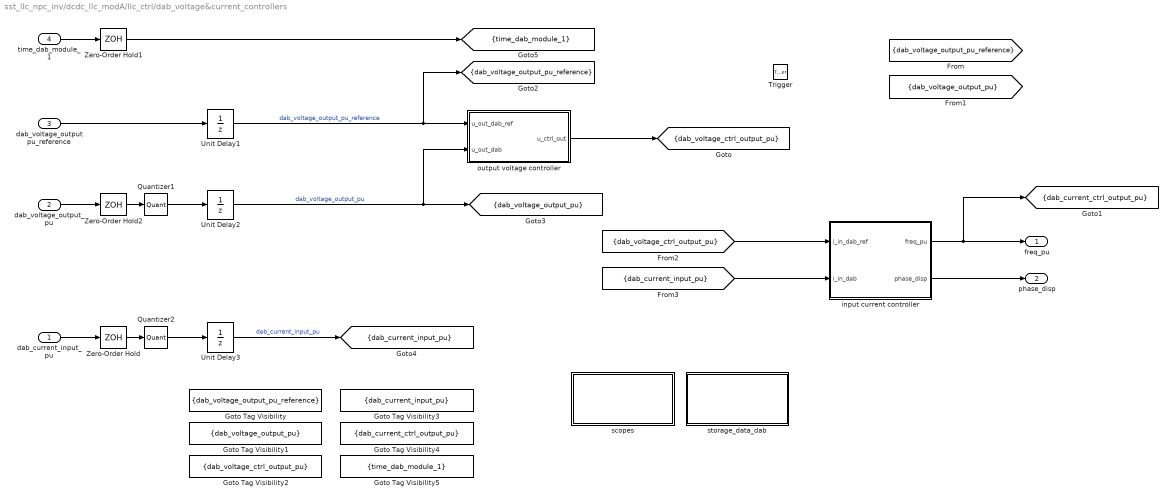
== system sst_llc_npc_inv/dcdc_llc_modA/llc_ctrl/dab_voltage&current_controllers ==
  dab_current_input_pu : Inport
  dab_voltage_output_pu : Inport  Port=2
  dab_voltage_output pu_reference : Inport  Port=3
  time_dab_module_1 : Inport  Port=4
  Trigger : TriggerPort  VariantControl=(inherit)  PortDimensions=1
  Goto Tag Visibility : GotoTagVisibility  GotoTag=dab_voltage_output_pu_reference
  Goto Tag Visibility1 : GotoTagVisibility  GotoTag=dab_voltage_output_pu
  Goto Tag Visibility2 : GotoTagVisibility  GotoTag=dab_voltage_ctrl_output_pu
  Goto Tag Visibility3 : GotoTagVisibility  GotoTag=dab_current_input_pu
  Goto Tag Visibility4 : GotoTagVisibility  GotoTag=dab_current_ctrl_output_pu
  Goto Tag Visibility5 : GotoTagVisibility  GotoTag=time_dab_module_1
  Quantizer1 : Quantizer  QuantizationInterval=adc12_quantization
  Quantizer2 : Quantizer  QuantizationInterval=adc12_quantization
  Unit Delay1 : UnitDelay  SampleTime=-1  HasFrameUpgradeWarning=on
  Unit Delay2 : UnitDelay  SampleTime=-1  HasFrameUpgradeWarning=on
  Unit Delay3 : UnitDelay  SampleTime=-1  HasFrameUpgradeWarning=on
  Zero-Order Hold : ZeroOrderHold  SampleTime=-1
  Zero-Order Hold1 : ZeroOrderHold  SampleTime=-1
  Zero-Order Hold2 : ZeroOrderHold  SampleTime=-1
  input current controller : Subsystem
  output voltage controller : Subsystem
  scopes : Subsystem
  storage_data_dab : Subsystem
  freq_pu : Outport
  phase_disp : Outport  Port=2
  tag scope: dab_current_ctrl_output_pu=scoped, dab_current_input_pu=scoped, dab_voltage_ctrl_output_pu=scoped, dab_voltage_output_pu=scoped, dab_voltage_output_pu_reference=scoped, time_dab_module_1=scoped
  wires:
  input current controller/1(freq_pu) -> freq_pu/1, [dab_current_ctrl_output_pu]
  output voltage controller/1(u_ctrl_out) -> [dab_voltage_ctrl_output_pu]
  dab_voltage_output_pu/1 -> Zero-Order Hold2/1
  dab_current_input_pu/1 -> Zero-Order Hold/1
  Unit Delay1/1 -> [dab_voltage_output_pu_reference], output voltage controller/1(u_out_dab_ref)  "dab_voltage_output_pu_reference"
  Unit Delay2/1 -> output voltage controller/2(u_out_dab), [dab_voltage_output_pu]  "dab_voltage_output_pu"
  Unit Delay3/1 -> [dab_current_input_pu]  "dab_current_input_pu"
  Zero-Order Hold/1 -> Quantizer2/1
  Zero-Order Hold2/1 -> Quantizer1/1
  dab_voltage_output pu_reference/1 -> Unit Delay1/1
  Quantizer1/1 -> Unit Delay2/1
  Quantizer2/1 -> Unit Delay3/1
  time_dab_module_1/1 -> Zero-Order Hold1/1
  Zero-Order Hold1/1 -> [time_dab_module_1]
  input current controller/2(phase_disp) -> phase_disp/1
  [dab_voltage_ctrl_output_pu] -> input current controller/1(i_in_dab_ref)
  [dab_current_input_pu] -> input current controller/2(i_in_dab)

== system sst_llc_npc_inv/dcdc_llc_modA/llc_ctrl/modulator ==
  freq_pu : Inport
  phase_displacement : Inport  Port=2
  Constant : Constant  Value=0.48
  resonant_llc_modulator : resonant_llc_modulator/resonant_llc_modulator  freq_base=fPWM_DAB  fres=fres  pos_cmd_gate=15  neg_cmd_gate=-10  tc=tc  trgo_double_update=0  max_phase_displacement=pi/2  freq_min=fPWM_DAB/5  freq_max=fPWM_DAB/2
  dab_gate_cmds : Outport
  tag scope: TRGO_DCDC_1=global
  wires:
  resonant_llc_modulator/2 -> [TRGO_DCDC_1]
  [time_dab_module_1] -> resonant_llc_modulator/3
  resonant_llc_modulator/1 -> dab_gate_cmds/1
  phase_displacement/1 -> resonant_llc_modulator/2
  Constant/1 -> resonant_llc_modulator/1

== system sst_llc_npc_inv/dcdc_llc_modA/llc_ctrl/references ==
  Rate Limiter : RateLimiter  RisingSlewLimit=Vdab2_dc_nom*10  FallingSlewLimit=-Vdab2_dc_nom*10  SampleTimeMode=inherited
  Vout_dc_nom : Step  Time=1e-3  After=Vdab2_dc_nom  SampleTime=0
  vout_ref : Outport
  wires:
  Vout_dc_nom/1 -> Rate Limiter/1
  Rate Limiter/1 -> vout_ref/1

== system sst_llc_npc_inv/dcdc_llc_modA/llc_ctrl/sampling_i_filter1 ==
  in : Inport
  1/Ti3 : Gain  Gain=1/Idc_FS  OutDataTypeStr=double  SaturateOnIntegerOverflow=on  ParamDataTypeStr=Inherit: Same as input
  out_pu : Outport
  wires:
  1/Ti3/1 -> out_pu/1
  in/1 -> 1/Ti3/1

== system sst_llc_npc_inv/dcdc_llc_modA/llc_ctrl/sampling_v_filter1 ==
  in : Inport
  1/Ti3 : Gain  Gain=1/Vdc_FS  OutDataTypeStr=double  SaturateOnIntegerOverflow=on  ParamDataTypeStr=Inherit: Same as input
  out_pu : Outport
  wires:
  1/Ti3/1 -> out_pu/1
  in/1 -> 1/Ti3/1

== system sst_llc_npc_inv/dcdc_llc_modA/llc_ctrl/sampling_v_filter2 ==
  in : Inport
  1/Ti3 : Gain  Gain=1/Vdc_FS  OutDataTypeStr=double  SaturateOnIntegerOverflow=on  ParamDataTypeStr=Inherit: Same as input
  Saturation : Saturate  UpperLimit=1  LowerLimit=0  OutDataTypeStr=double
  out_pu : Outport
  wires:
  Saturation/1 -> out_pu/1
  1/Ti3/1 -> Saturation/1
  in/1 -> 1/Ti3/1

== system sst_llc_npc_inv/dcdc_llc_modB/dc//dc with galvanic isolation/full-bridge 1 ==
  gate_commands : Inport
  full-bridge ideal switch based : full_bridge_ideal_switch/full-bridge ideal switch based  Rds_on=dab.Rds_on  Vdon_diode=dab.Vdon_diode  Rdon_diode=dab.Rdon_diode  Csnubber=dab.Csnubber  Rsnubber=dab.Rsnubber  Vth=7.5
  uac_1(+) : PMIOPort  Side=Left
  uac_1(-) : PMIOPort  Port=2  Side=Left
  Udc(+) : PMIOPort  Port=3  Side=Right
  Udc(-) : PMIOPort  Port=4  Side=Right
  wires:
  gate_commands/1 -> full-bridge ideal switch based/1
  connections:
  full-bridge ideal switch based/LConn1 -- Udc(+)/RConn1
  full-bridge ideal switch based/LConn2 -- Udc(-)/RConn1
  full-bridge ideal switch based/RConn2 -- uac_1(-)/RConn1
  full-bridge ideal switch based/RConn1 -- uac_1(+)/RConn1

== system sst_llc_npc_inv/dcdc_llc_modB/dc//dc with galvanic isolation/full-bridge 2 ==
  gate_commands : Inport
  CFi_dc2 : fl_lib/Electrical/Electrical Elements/Capacitor  c=CFi_dc2 F  r=RCFi_dc2_internal Ohm  g=0 1/Ohm  i_specify=off  i_priority=None  i=0 A  i_nominal_specify=off  i_nominal_value=1  i_nominal_unit=A  v_specify=off  v_priority=None  v=0 V  v_nominal_specify=off  v_nominal_value=1  v_nominal_unit=V  vc_specify=off  vc_priority=High  vc=0 V  vc_nominal_specify=off  vc_nominal_value=1  vc_nominal_unit=V
  Current Sensor2 : fl_lib/Electrical/Electrical Sensors/Current Sensor
  PS-Simulink Converter6 : nesl_utility/PS-Simulink Converter  PhysicalDomain=network_engine_domain  SubClassName=ps_output  LeftPortType=input  RightPortType=output  PseudoPeriodic=off  Frequencies=[]  VectorFormat=1-D array  Unit=A  AffineConversion=on
  full-bridge ideal switch based : full_bridge_ideal_switch/full-bridge ideal switch based  Rds_on=dab.Rds_on  Vdon_diode=dab.Vdon_diode  Rdon_diode=dab.Rdon_diode  Csnubber=dab.Csnubber  Rsnubber=dab.Rsnubber  Vth=7.5
  uac_2(+) : PMIOPort  Side=Left
  uac_2(-) : PMIOPort  Port=2  Side=Left
  udc(+) : PMIOPort  Port=3  Side=Right
  udc(-) : PMIOPort  Port=4  Side=Right
  tag scope: CFi_dc2_current_modB=global
  wires:
  PS-Simulink Converter6/1 -> [CFi_dc2_current_modB]  "CFi_dc2_current_modA"
  gate_commands/1 -> full-bridge ideal switch based/1
  connections:
  full-bridge ideal switch based/RConn2 -- uac_2(-)/RConn1
  full-bridge ideal switch based/RConn1 -- uac_2(+)/RConn1
  CFi_dc2/RConn1 -- Current Sensor2/LConn1
  PS-Simulink Converter6/LConn1 -- Current Sensor2/RConn1
  udc(-)/RConn1 -- full-bridge ideal switch based/LConn2 -- Current Sensor2/RConn2
  CFi_dc2/LConn1 -- full-bridge ideal switch based/LConn1 -- udc(+)/RConn1

== system sst_llc_npc_inv/dcdc_llc_modB/dc//dc with galvanic isolation/single_phase_dab_transformer ==
  Capacitor : fl_lib/Electrical/Electrical Elements/Capacitor  c=Cs1 F  r=1e-6 Ohm  g=0 1/Ohm  i_specify=off  i_priority=None  i=0 A  i_nominal_specify=off  i_nominal_value=1  i_nominal_unit=A  v_specify=off  v_priority=None  v=0 V  v_nominal_specify=off  v_nominal_value=1  v_nominal_unit=V  vc_specify=off  vc_priority=High  vc=0 V  vc_nominal_specify=off  vc_nominal_value=1  vc_nominal_unit=V
  Capacitor1 : fl_lib/Electrical/Electrical Elements/Capacitor  c=Cs2 F  r=1e-6 Ohm  g=0 1/Ohm  i_specify=off  i_priority=None  i=0 A  i_nominal_specify=off  i_nominal_value=1  i_nominal_unit=A  v_specify=off  v_priority=None  v=0 V  v_nominal_specify=off  v_nominal_value=1  v_nominal_unit=V  vc_specify=off  vc_priority=High  vc=0 V  vc_nominal_specify=off  vc_nominal_value=1  vc_nominal_unit=V
  Current Sensor : fl_lib/Electrical/Electrical Sensors/Current Sensor
  Current Sensor1 : fl_lib/Electrical/Electrical Sensors/Current Sensor
  Voltage Sensor1 : fl_lib/Electrical/Electrical Sensors/Voltage Sensor
  Voltage Sensor3 : fl_lib/Electrical/Electrical Sensors/Voltage Sensor
  i1_dab_transformer : nesl_utility/PS-Simulink Converter  PhysicalDomain=network_engine_domain  SubClassName=ps_output  LeftPortType=input  RightPortType=output  PseudoPeriodic=off  Frequencies=[]  VectorFormat=1-D array  Unit=A  AffineConversion=off
  i2_dab_transformer : nesl_utility/PS-Simulink Converter  PhysicalDomain=network_engine_domain  SubClassName=ps_output  LeftPortType=input  RightPortType=output  PseudoPeriodic=off  Frequencies=[]  VectorFormat=1-D array  Unit=A  AffineConversion=off
  single_phase_transformer : single_phase_transformer/single_phase_transformer  lm_trafo=lm_trafo  m1=m1  m2=m2  rd1_trafo=rd1_trafo  rd2_trafo=rd2_trafo  ld1_trafo=ld1_trafo  ld2_trafo=ld2_trafo  rfe_trafo=rfe_trafo  length_core=0.5  mu0=1.256637e-6  mur=70
  single_phase_transformer - scope : Scope
      settings: ActiveDisplayYMinimum=-1507.7800736606021  ActiveDisplayYMaximum=1558.2525629015804  DataLoggingVariableName=ScopeData21
  u1_dab_transformer : nesl_utility/PS-Simulink Converter  PhysicalDomain=network_engine_domain  SubClassName=ps_output  LeftPortType=input  RightPortType=output  PseudoPeriodic=off  Frequencies=[]  VectorFormat=1-D array  Unit=V  AffineConversion=on
  u2_dab_transformer : nesl_utility/PS-Simulink Converter  PhysicalDomain=network_engine_domain  SubClassName=ps_output  LeftPortType=input  RightPortType=output  PseudoPeriodic=off  Frequencies=[]  VectorFormat=1-D array  Unit=V  AffineConversion=on
  u1(+) : PMIOPort  Side=Left
  u2(+) : PMIOPort  Port=2  Side=Right
  u1(-) : PMIOPort  Port=3  Side=Left
  u2(-) : PMIOPort  Port=4  Side=Right
  tag scope: i1_dab_transformer_modB=global, i2_dab_transformer_modB=global, u1_dab_transformer_modB=global, u2_dab_transformer_modB=global
  wires:
  single_phase_transformer/1 -> single_phase_transformer - scope/1
  i1_dab_transformer/1 -> [i1_dab_transformer_modB]
  u1_dab_transformer/1 -> [u1_dab_transformer_modB]
  u2_dab_transformer/1 -> [u2_dab_transformer_modB]
  i2_dab_transformer/1 -> [i2_dab_transformer_modB]
  connections:
  single_phase_transformer/RConn1 -- Capacitor1/LConn1
  Capacitor/LConn1 -- Current Sensor1/RConn2
  single_phase_transformer/LConn1 -- Capacitor/RConn1
  Current Sensor/LConn1 -- Capacitor1/RConn1 -- Voltage Sensor3/LConn1
  Current Sensor1/RConn1 -- i1_dab_transformer/LConn1
  Voltage Sensor1/RConn1 -- u1_dab_transformer/LConn1
  u1(+)/RConn1 -- Voltage Sensor1/LConn1 -- Current Sensor1/LConn1
  Voltage Sensor1/RConn2 -- single_phase_transformer/LConn2 -- u1(-)/RConn1
  Voltage Sensor3/RConn1 -- u2_dab_transformer/LConn1
  Current Sensor/RConn1 -- i2_dab_transformer/LConn1
  u2(-)/RConn1 -- single_phase_transformer/RConn2 -- Voltage Sensor3/RConn2
  Current Sensor/RConn2 -- u2(+)/RConn1
